simulink model "doblependulompat"  (R2013a)
settings: Solver=ode23s  StartTime=0.0  StopTime=10  RelTol=1e-3
values from neighbouring files (symbols this model uses):
  g = 9.81    [miosinlazoalgebraico.m]    (also in yovalores.m)
  theta1 = (m1*lc1*lc1)+(m2*l1*l1)+I1    (= 0.09775488)    [miosinlazoalgebraico.m]
  theta2 = (m2*lc2*lc2)+I2    (= 0.00775807)    [miosinlazoalgebraico.m]
  theta3 = (m2*l1*l2)    (= 0.0287)    [miosinlazoalgebraico.m]
  theta4 = (m1*lc1)+(m2*l1)    (= 0.495148)    [miosinlazoalgebraico.m]
  theta5 = (m2*lc2)    (= 0.044485)    [miosinlazoalgebraico.m]
settings Model: Creator=Daniel  LastModifiedBy=Daniel
settings DebuggingCC: ConsistencyChecking=warning  AlgebraicLoopMsg=none  ArtificialAlgebraicLoopMsg=none  SolverPrmCheckMsg=none

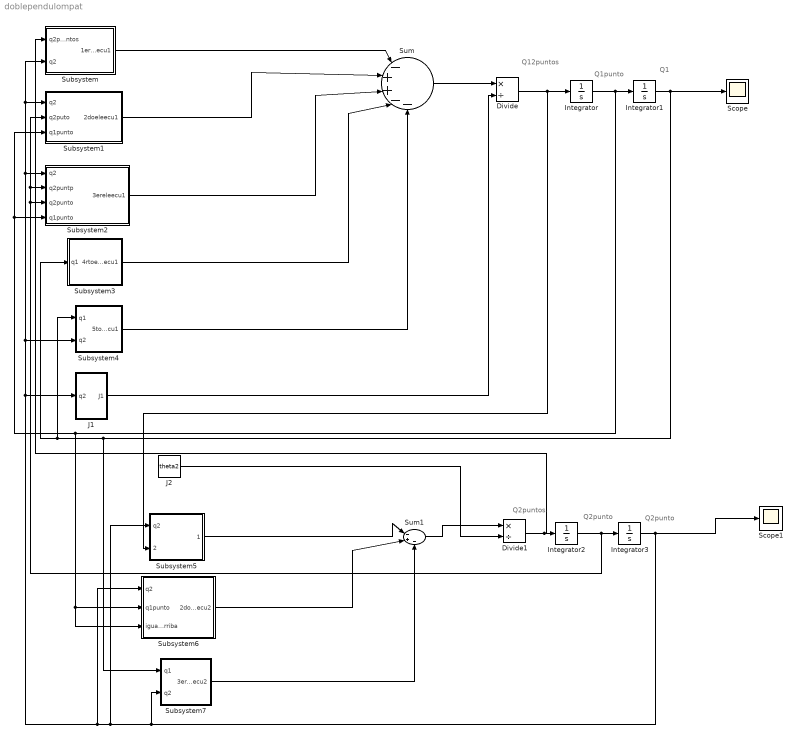
== system doblependulompat ==
  note: Q2punto
  note: Q2punto
  note: Q2puntos
  note: Q1
  note: Q1punto
  note: Q12puntos
  Divide : Product  Inputs=*/
  Divide1 : Product  Inputs=*/
  Integrator : Integrator
  Integrator1 : Integrator  InitialCondition=-pi/2
  Integrator2 : Integrator
  Integrator3 : Integrator  InitialCondition=-pi/2
  J1 : Subsystem
  J2 : Constant  Value=theta2
  Scope : Scope
      settings: YMin=2.73642  YMax=2.7365
  Scope1 : Scope
  Subsystem : Subsystem
  Subsystem1 : Subsystem
  Subsystem2 : Subsystem
  Subsystem3 : Subsystem
  Subsystem4 : Subsystem
  Subsystem5 : Subsystem
  Subsystem6 : Subsystem
  Subsystem7 : Subsystem
  Sum : Sum  Inputs=|-++--
  Sum1 : Sum  Inputs=|-+-
  wires:
  Subsystem/1(1ereleecu1) -> Sum/1
  Subsystem1/1(2doeleecu1) -> Sum/2
  Subsystem2/1(3ereleecu1) -> Sum/3
  Subsystem3/1(4rtoeleecu1) -> Sum/4
  Subsystem4/1(5toeleecu1) -> Sum/5
  Sum/1 -> Divide/1
  J1/1(J1) -> Divide/2
  Subsystem5/1(1ereleecu2) -> Sum1/1
  Subsystem6/1(2doeleecu2) -> Sum1/2
  Subsystem7/1(3ereleecu2) -> Sum1/3
  Sum1/1 -> Divide1/1
  J2/1 -> Divide1/2
  Divide1/1 -> Subsystem/1(q2puntos), Integrator2/1
  Integrator2/1 -> Subsystem2/3(q2punto), Subsystem2/2(q2puntp), Subsystem1/2(q2puto), Integrator3/1
  Divide/1 -> Subsystem5/2(q1dospuntos), Integrator/1
  Integrator/1 -> Subsystem6/3(igualq,arriba), Subsystem6/2(q1punto), Subsystem2/4(q1punto), Subsystem1/3(q1punto), Integrator1/1
  Integrator3/1 -> Scope1/1, Subsystem7/2(q2), Subsystem5/1(q2), Subsystem6/1(q2), J1/1(q2), Subsystem4/2(q2), Subsystem2/1(q2), Subsystem1/1(q2), Subsystem/2(q2)
  Integrator1/1 -> Scope/1, Subsystem7/1(q1), Subsystem4/1(q1), Subsystem3/1(q1)

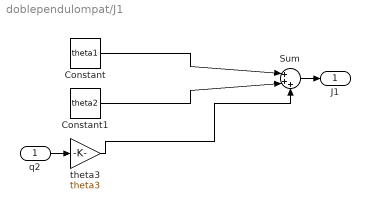
== system doblependulompat/J1 ==
  q2 : Inport
  Constant : Constant  Value=theta1
  Constant1 : Constant  Value=theta2
  Sum : Sum  Inputs=|+++
  theta3 : Gain  Gain=theta3
  J1 : Outport
  wires:
  Constant/1 -> Sum/1
  Constant1/1 -> Sum/2
  theta3/1 -> Sum/3
  Sum/1 -> J1/1
  q2/1 -> theta3/1

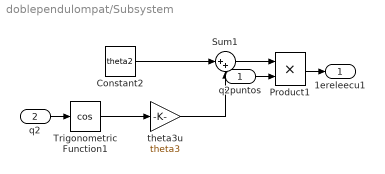
== system doblependulompat/Subsystem ==
  q2puntos : Inport
  q2 : Inport  Port=2
  Constant2 : Constant  Value=theta2
  Product1 : Product
  Sum1 : Sum  Inputs=|++
  Trigonometric Function1 : Trigonometry  Operator=cos
  theta3u : Gain  Gain=theta3
  1ereleecu1 : Outport
  wires:
  Constant2/1 -> Sum1/1
  theta3u/1 -> Sum1/2
  Trigonometric Function1/1 -> theta3u/1
  Sum1/1 -> Product1/1
  q2puntos/1 -> Product1/2
  q2/1 -> Trigonometric Function1/1
  Product1/1 -> 1ereleecu1/1

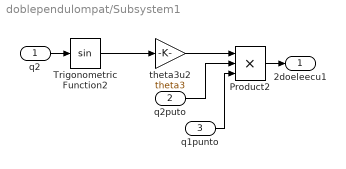
== system doblependulompat/Subsystem1 ==
  q2 : Inport
  q2puto : Inport  Port=2
  q1punto : Inport  Port=3
  Product2 : Product  Inputs=3
  Trigonometric Function2 : Trigonometry
  theta3u2 : Gain  Gain=theta3
  2doeleecu1 : Outport
  wires:
  Trigonometric Function2/1 -> theta3u2/1
  theta3u2/1 -> Product2/1
  q2/1 -> Trigonometric Function2/1
  q1punto/1 -> Product2/3
  q2puto/1 -> Product2/2
  Product2/1 -> 2doeleecu1/1

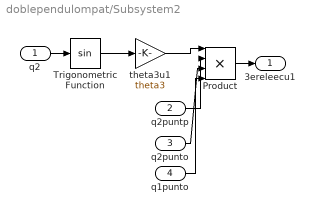
== system doblependulompat/Subsystem2 ==
  q2 : Inport
  q2puntp : Inport  Port=2
  q2punto : Inport  Port=3
  q1punto : Inport  Port=4
  Product : Product  Inputs=4
  Trigonometric Function : Trigonometry
  theta3u1 : Gain  Gain=theta3
  3ereleecu1 : Outport
  wires:
  q2/1 -> Trigonometric Function/1
  q2puntp/1 -> Product/2
  q2punto/1 -> Product/3
  q1punto/1 -> Product/4
  Product/1 -> 3ereleecu1/1
  Trigonometric Function/1 -> theta3u1/1
  theta3u1/1 -> Product/1

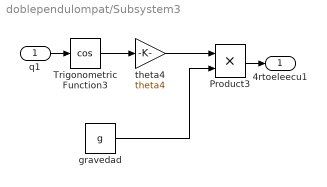
== system doblependulompat/Subsystem3 ==
  q1 : Inport
  Product3 : Product
  Trigonometric Function3 : Trigonometry  Operator=cos
  gravedad : Constant  Value=g
  theta4 : Gain  Gain=theta4
  4rtoeleecu1 : Outport
  wires:
  Product3/1 -> 4rtoeleecu1/1
  q1/1 -> Trigonometric Function3/1
  Trigonometric Function3/1 -> theta4/1
  theta4/1 -> Product3/1
  gravedad/1 -> Product3/2

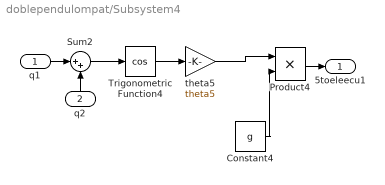
== system doblependulompat/Subsystem4 ==
  q1 : Inport
  q2 : Inport  Port=2
  Constant4 : Constant  Value=g
  Product4 : Product
  Sum2 : Sum  Inputs=|++
  Trigonometric Function4 : Trigonometry  Operator=cos
  theta5 : Gain  Gain=theta5
  5toeleecu1 : Outport
  wires:
  q1/1 -> Sum2/1
  Product4/1 -> 5toeleecu1/1
  q2/1 -> Sum2/2
  Trigonometric Function4/1 -> theta5/1
  Sum2/1 -> Trigonometric Function4/1
  theta5/1 -> Product4/1
  Constant4/1 -> Product4/2

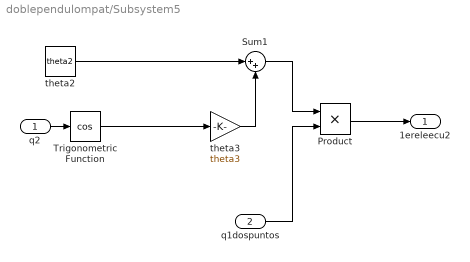
== system doblependulompat/Subsystem5 ==
  q2 : Inport
  q1dospuntos : Inport  Port=2
  Product : Product
  Sum1 : Sum  Inputs=|++
  Trigonometric Function : Trigonometry  Operator=cos
  theta2 : Constant  Value=theta2
  theta3 : Gain  Gain=theta3
  1ereleecu2 : Outport
  wires:
  Trigonometric Function/1 -> theta3/1
  theta2/1 -> Sum1/1
  theta3/1 -> Sum1/2
  q2/1 -> Trigonometric Function/1
  Sum1/1 -> Product/1
  q1dospuntos/1 -> Product/2
  Product/1 -> 1ereleecu2/1

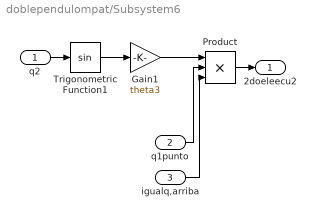
== system doblependulompat/Subsystem6 ==
  q2 : Inport
  q1punto : Inport  Port=2
  igualq,arriba : Inport  Port=3
  Gain1 : Gain  Gain=theta3
  Product : Product  Inputs=3
  Trigonometric Function1 : Trigonometry
  2doeleecu2 : Outport
  wires:
  Trigonometric Function1/1 -> Gain1/1
  Product/1 -> 2doeleecu2/1
  q2/1 -> Trigonometric Function1/1
  igualq,arriba/1 -> Product/3
  q1punto/1 -> Product/2
  Gain1/1 -> Product/1

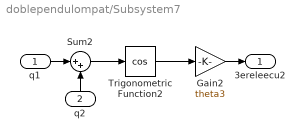
== system doblependulompat/Subsystem7 ==
  q1 : Inport
  q2 : Inport  Port=2
  Gain2 : Gain  Gain=theta3
  Sum2 : Sum  Inputs=|++
  Trigonometric Function2 : Trigonometry  Operator=cos
  3ereleecu2 : Outport
  wires:
  Gain2/1 -> 3ereleecu2/1
  q1/1 -> Sum2/1
  Trigonometric Function2/1 -> Gain2/1
  Sum2/1 -> Trigonometric Function2/1
  q2/1 -> Sum2/2
